simulink model "serialArduinoRobotHand"  (R2022a)
settings: Solver=VariableStepAuto  StartTime=0.0  StopTime=inf  RelTol=1e-3
undefined symbols (not defined in the file): Serial_Port, Standard_Devices
libraries: sldrtlib x2
settings Model: SimulationMode=accelerator  Creator=lunde  LastModifiedBy=lunde

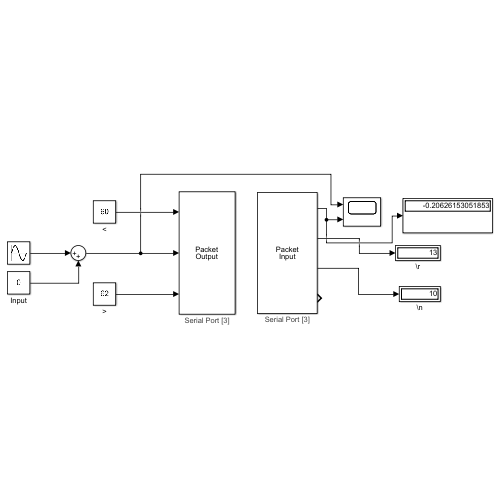
[thumbnail: Simulink's stored preview of the top-level diagram]
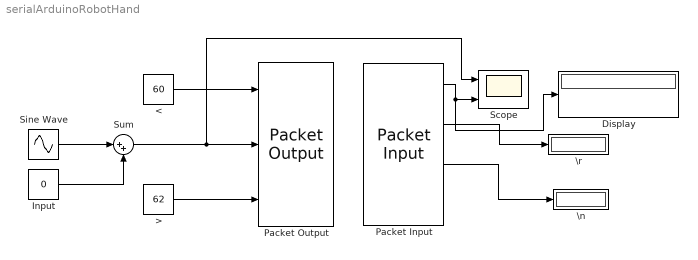
== system serialArduinoRobotHand ==
  < : Constant  Value=60
  > : Constant  Value=62
  Display : Display
      settings: Format=decimal (Stored Integer)
  Input : Constant  Value=0  OutDataTypeStr=single
  Packet Input : sldrtlib/Packet Input  SampleTime=0.1  MaxMissedTicks=1000  ShowMissedTicks=off  YieldWhenWaiting=off  DrvName=Standard_Devices/Serial_Port  DrvAddress=3  DrvOptions=[9600 8 0 0 0 0 0 0]  PacketSize=6  DataTypes={'1*single', '1*uint8', '1*uint8'}  ShowReady=on  ShowError=off  PacketID=1  ByteOrder=1  ShowTimestamp=off
      settings: AttributesFormatString=Serial Port [3]
  Packet Output : sldrtlib/Packet Output  SampleTime=0.1  MaxMissedTicks=1000  ShowMissedTicks=off  YieldWhenWaiting=off  DrvName=Standard_Devices/Serial_Port  DrvAddress=3  DrvOptions=[9600 8 0 0 0 0 0 0]  PacketSize=6  DataTypes={'1*uint8', '1*single', '1*uint8'}  ShowReady=off  ShowError=off  PacketID=1  ByteOrder=1  InitialValue=[]  FinalValue=[]
      settings: AttributesFormatString=Serial Port [3]
  Scope : Scope  NumInputPorts=2
  Sine Wave : Sin  Amplitude=0.5  Frequency=0.5  SampleTime=0
  Sum : Sum  Inputs=|++  AccumDataTypeStr=single  OutDataTypeStr=single  RndMeth=Nearest
  \n : Display
      settings: Format=decimal (Stored Integer)
  \r : Display
      settings: Format=decimal (Stored Integer)
  wires:
  Packet Input/1 -> Scope/2, Display/1
  </1 -> Packet Output/1
  >/1 -> Packet Output/3
  Packet Input/3 -> \n/1
  Packet Input/2 -> \r/1
  Sine Wave/1 -> Sum/1
  Input/1 -> Sum/2
  Sum/1 -> Scope/1, Packet Output/2
